simulink subsystem "Next_waypoints_array"  (R2022b)
settings: Solver=VariableStepAuto  StartTime=0.0  StopTime=10.0  RelTol=1e-3
libraries: CarMaker4SL x3
settings Model: Creator=user  LastModifiedBy=user

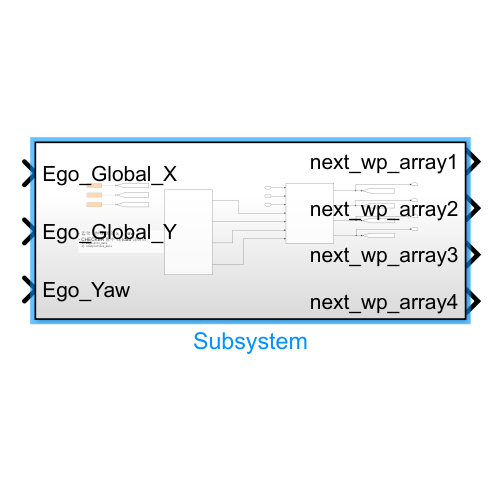
[thumbnail: Simulink's stored preview of the top-level diagram]
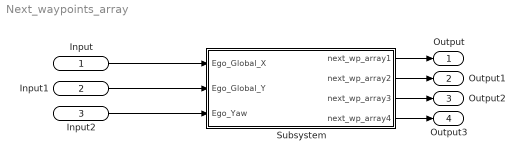
== system Next_waypoints_array ==
  Input : Inport
  Input1 : Inport  Port=2
  Input2 : Inport  Port=3
  Subsystem : Subsystem
  Output : Outport
  Output1 : Outport  Port=2
  Output2 : Outport  Port=3
  Output3 : Outport  Port=4
  wires:
  Input/1 -> Subsystem/1(Ego_Global_X)
  Input1/1 -> Subsystem/2(Ego_Global_Y)
  Input2/1 -> Subsystem/3(Ego_Yaw)
  Subsystem/1(next_wp_array1) -> Output/1
  Subsystem/2(next_wp_array2) -> Output1/1
  Subsystem/3(next_wp_array3) -> Output2/1
  Subsystem/4(next_wp_array4) -> Output3/1

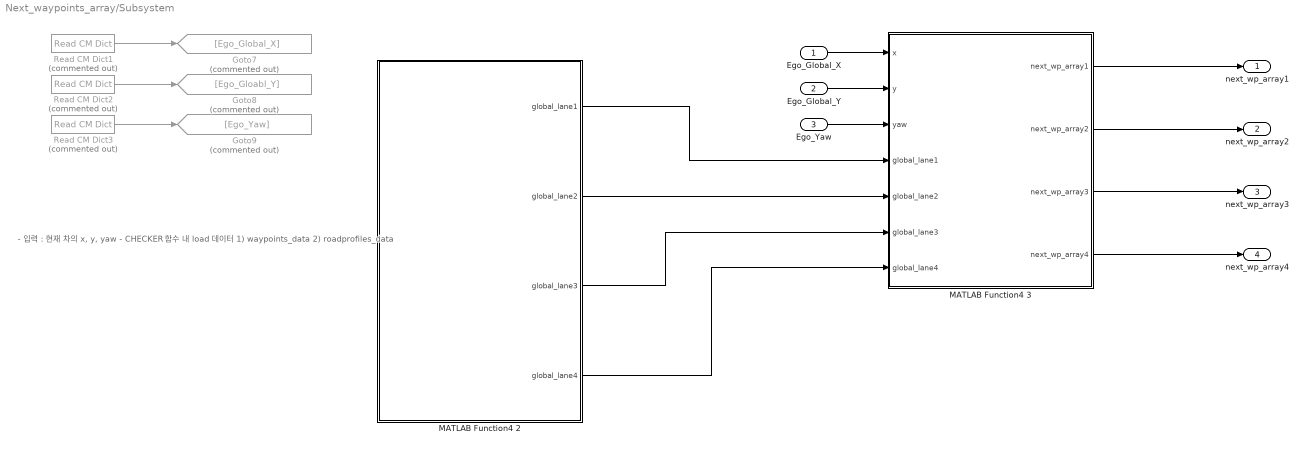
== system Next_waypoints_array/Subsystem ==
  note: - 입력 : 현재 차의 x, y, yaw
      | - CHECKER 함수 내 load 데이터
      | 1) waypoints_data
      | 2) roadprofiles_data
  Ego_Global_X : Inport
  Ego_Global_Y : Inport  Port=2
  Ego_Yaw : Inport  Port=3
  Goto7 : Goto  Commented=on  GotoTag=Ego_Global_X
  Goto8 : Goto  Commented=on  GotoTag=Ego_Gloabl_Y
  Goto9 : Goto  Commented=on  GotoTag=Ego_Yaw
  MATLAB Function4 2 : MATLAB Function  TreatAsAtomicUnit=on
  MATLAB Function4 3 : MATLAB Function  TreatAsAtomicUnit=on
  Read CM Dict1 : CarMaker4SL/Read CM Dict  Commented=on  xname=Car.Fr1.tx  xsync=off  xstime=Inherited
  Read CM Dict2 : CarMaker4SL/Read CM Dict  Commented=on  xname=Car.Fr1.ty  xsync=off  xstime=Inherited
  Read CM Dict3 : CarMaker4SL/Read CM Dict  Commented=on  xname=Car.Fr1.rz  xsync=off  xstime=Inherited
  next_wp_array1 : Outport
  next_wp_array2 : Outport  Port=2
  next_wp_array3 : Outport  Port=3
  next_wp_array4 : Outport  Port=4
  wires:
  MATLAB Function4 2/4(global_lane4) -> MATLAB Function4 3/7(global_lane4)
  MATLAB Function4 2/3(global_lane3) -> MATLAB Function4 3/6(global_lane3)
  MATLAB Function4 3/4(next_wp_array4) -> next_wp_array4/1
  MATLAB Function4 2/2(global_lane2) -> MATLAB Function4 3/5(global_lane2)
  MATLAB Function4 3/3(next_wp_array3) -> next_wp_array3/1
  Read CM Dict2/1 -> Goto8/1
  Read CM Dict3/1 -> Goto9/1
  Read CM Dict1/1 -> Goto7/1
  MATLAB Function4 3/2(next_wp_array2) -> next_wp_array2/1
  MATLAB Function4 3/1(next_wp_array1) -> next_wp_array1/1
  MATLAB Function4 2/1(global_lane1) -> MATLAB Function4 3/4(global_lane1)
  Ego_Global_X/1 -> MATLAB Function4 3/1(x)
  Ego_Global_Y/1 -> MATLAB Function4 3/2(y)
  Ego_Yaw/1 -> MATLAB Function4 3/3(yaw)

== matlab function Next_waypoints_array/Subsystem/MATLAB Function4 2 ==
  settings: sampleTime=0.1
  data: global_lane1 output; global_lane2 output; global_lane3 output; global_lane4 output
function [global_lane1, global_lane2, global_lane3, global_lane4] = CHECKER()

    %% Localization plotter
    f1 = load('waypoints_data.mat');
    f2 = load('roadprofiles_data.mat');

    n_waypoint = height(f1.ids);
    n_roadprofile = height(f2.ids);

    % 미리 고정된 크기의 큰 배열로 초기화
    max_size = 1000; % 필요에 따라 적절한 값으로 설정
    global_lane1 = NaN(max_size, 2); % NaN으로 초기화하여 미리 고정 크기를 설정
    global_lane2 = NaN(max_size, 2);
    global_lane3 = NaN(max_size, 2);
    global_lane4 = NaN(max_size, 2);

    lane1_idx = 1;
    lane2_idx = 1;
    lane3_idx = 1;
    lane4_idx = 1;

    % Loop through each road profile
    for i = 1 : n_roadprofile
        x = zeros(1, 50);
        y = zeros(1, 50);
        idx = 1;

        for j = 1:50
            if f2.waypoints(i,j) ~= 0
                x(idx) = f1.waypoints(f2.waypoints(i,j),1);
                y(idx) = f1.waypoints(f2.waypoints(i,j),2);

                if x(idx) >= -200 && x(idx) <= 200 && y(idx) >= -200 && y(idx) <= 200
                    idx = idx + 1;
                end
            end
        end

        % 유효한 값을 각 lane에 추가
        if ismember(i, 1:10)
            global_lane1(lane1_idx:lane1_idx+idx-2, :) = [x(1:idx-1)', y(1:idx-1)'];
            lane1_idx = lane1_idx + idx - 1;
        elseif ismember(i, 11:20)
            global_lane2(lane2_idx:lane2_idx+idx-2, :) = [x(1:idx-1)', y(1:idx-1)'];
            lane2_idx = lane2_idx + idx - 1;
        elseif ismember(i, 21:30)
            global_lane3(lane3_idx:lane3_idx+idx-2, :) = [x(1:idx-1)', y(1:idx-1)'];
            lane3_idx = lane3_idx + idx - 1;
        elseif ismember(i, 31:33)
            global_lane4(lane4_idx:lane4_idx+idx-2, :) = [x(1:idx-1)', y(1:idx-1)'];
            lane4_idx = lane4_idx + idx - 1;
        end
    end

    % 더 이상 할당할 필요 없이 global_lane을 그대로 사용
end

== matlab function Next_waypoints_array/Subsystem/MATLAB Function4 3 ==
  settings: sampleTime=0.1
  data: x input; y input; next_wp_array1 output; yaw input; next_wp_array2 output; next_wp_array3 output; next_wp_array4 output; global_lane1 input; global_lane2 input; global_lane3 input; global_lane4 input
function [next_wp_array1, next_wp_array2, next_wp_array3, next_wp_array4] = next_waypoint(x, y, yaw, global_lane1, global_lane2, global_lane3, global_lane4)
    %parameter setting
    distance = 2; num_wp = 10; %distance : waypoints사이 거리, num_wp : waypoints 개수
    limit_dist = (num_wp * distance) / 2; %limit_dist : limit_dist이내에서만 waypoints저장

    waypoints1 = global_lane1; % Use only lane 1 waypoints
    waypoints2 = global_lane2;
    waypoints3 = global_lane3;
    waypoints4 = global_lane4;

    % Initialize output variables with 1x1 size
    closest_wp_idx1 = 0;
    closest_wp_idx2 = 0;
    closest_wp_idx3 = 0;
    closest_wp_idx4 = 0;
    distances1 = 0;
    distances2 = 0;
    distances3 = 0;
    distances4 = 0;

    % Initialize the next waypoints array
    next_wp_array1 = nan(num_wp, 2); % 초기값을 NaN으로 설정하여 25 이상의 거리인 경우 생략
    next_wp_array2 = nan(num_wp, 2);
    next_wp_array3 = nan(num_wp, 2);
    next_wp_array4 = nan(num_wp, 2);
    
    % Start from the current position
    %current_pos = [x, y];
    current_pos_x = x;
    current_pos_y = y;
%     % Find the closest waypoint index based on current position and yaw
%     [closest_wp_idx1, closest_wp_idx2, closest_wp_idx3, closest_wp_idx4] = find_nearest_waypoint(current_pos(1), current_pos(2), yaw);
    distances1 = sqrt((global_lane1(:, 1) - current_pos_x).^2 + (global_lane1(:, 2) - current_pos_y).^2);
    distances2 = sqrt((global_lane2(:, 1) - current_pos_x).^2 + (global_lane2(:, 2) - current_pos_y).^2);
    distances3 = sqrt((global_lane3(:, 1) - current_pos_x).^2 + (global_lane3(:, 2) - current_pos_y).^2);
    distances4 = sqrt((global_lane4(:, 1) - current_pos_x).^2 + (global_lane4(:, 2) - current_pos_y).^2);
    [~, closest_wp_idx1] = min(distances1);
    [~, closest_wp_idx2] = min(distances2);
    [~, closest_wp_idx3] = min(distances3);
    [~, closest_wp_idx4] = min(distances4);

    % Ensure closest_wp_idx is within the range of global_lane1
    closest_wp_idx1 = mod(closest_wp_idx1 - 1, size(waypoints1, 1)) + 1; % Wrap around if out of bounds
    closest_wp_idx2 = mod(closest_wp_idx2 - 1, size(waypoints2, 1)) + 1; % Wrap around if out of bounds
    closest_wp_idx3 = mod(closest_wp_idx3- 1, size(waypoints3, 1)) + 1; % Wrap around if out of bounds
    closest_wp_idx4 = mod(closest_wp_idx4 - 1, size(waypoints4, 1)) + 1; % Wrap around if out of bounds

    % Loop to find next waypoints
    for i = 1:num_wp
        % Calculate the next position based on yaw and distance
        current_pos_x = current_pos_x + distance * cosd(yaw);
        current_pos_y = current_pos_y + distance * sind(yaw);

%       % Update the closest waypoint index based on the new position
%       [closest_wp_idx1, closest_wp_idx2, closest_wp_idx3, closest_wp_idx4] = find_nearest_waypoint(current_pos(1), current_pos(2), yaw);
        distances1 = sqrt((global_lane1(:, 1) - current_pos_x).^2 + (global_lane1(:, 2) - current_pos_y).^2);
        distances2 = sqrt((global_lane2(:, 1) - current_pos_x).^2 + (global_lane2(:, 2) - current_pos_y).^2);
        distances3 = sqrt((global_lane3(:, 1) - current_pos_x).^2 + (global_lane3(:, 2) - current_pos_y).^2);
        distances4 = sqrt((global_lane4(:, 1) - current_pos_x).^2 + (global_lane4(:, 2) - current_pos_y).^2);
        [~, closest_wp_idx1] = min(distances1);
        [~, closest_wp_idx2] = min(distances2);
        [~, closest_wp_idx3] = min(distances3);
        [~, closest_wp_idx4] = min(distances4);

        % Ensure closest_wp_idx is within the range of global_lane1
        closest_wp_idx1 = mod(closest_wp_idx1 - 1, size(waypoints1, 1)) + 1; % Wrap around if out of bounds
        closest_wp_idx2 = mod(closest_wp_idx2 - 1, size(waypoints2, 1)) + 1; % Wrap around if out of bounds
        closest_wp_idx3 = mod(closest_wp_idx3 - 1, size(waypoints3, 1)) + 1; % Wrap around if out of bounds
        closest_wp_idx4 = mod(closest_wp_idx4 - 1, size(waypoints4, 1)) + 1; % Wrap around if out of bounds
        
        % Store the next waypoint coordinates if distance <= limit_dist
        if distances1(closest_wp_idx1) <= limit_dist
            next_wp_array1(i, :) = waypoints1(closest_wp_idx1, :);
        end
        if distances2(closest_wp_idx2) <= limit_dist
            next_wp_array2(i, :) = waypoints2(closest_wp_idx2, :);
        end
        if distances3(closest_wp_idx3) <= limit_dist
            next_wp_array3(i, :) = waypoints3(closest_wp_idx3, :);
        end
        if distances4(closest_wp_idx4) <= limit_dist
            next_wp_array4(i, :) = waypoints4(closest_wp_idx4, :);
        end

    end
    
    
end
